simulink model "battery_pack"  (R2021a)
settings: Solver=VariableStepAuto  StartTime=0.0  StopTime=300  RelTol=1e-3
libraries: fl_lib x3, nesl_utility x3
settings Model: Creator=miche  LastModifiedBy=miche

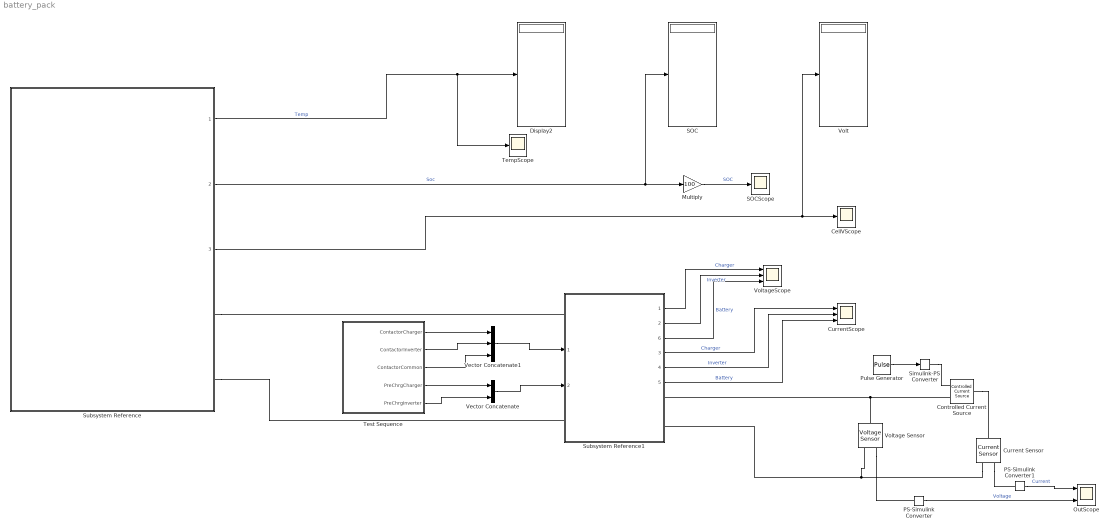
== system battery_pack ==
  CellVScope : Scope
  Controlled Current Source : fl_lib/Electrical/Electrical Sources/Controlled Current Source
  Current Sensor : fl_lib/Electrical/Electrical Sensors/Current Sensor
  CurrentScope : Scope  NumInputPorts=3
  Display2 : Display
  Multiply : Gain  Gain=100
  OutScope : Scope  NumInputPorts=2
  PS-Simulink Converter : nesl_utility/PS-Simulink Converter  PhysicalDomain=network_engine_domain  SubClassName=ps_output  LeftPortType=input  RightPortType=output  PseudoPeriodic=off  Frequencies=[]  Unit=inherit  AffineConversion=off
      settings: SourceProductBaseCode=PW,SS
  PS-Simulink Converter1 : nesl_utility/PS-Simulink Converter  PhysicalDomain=network_engine_domain  SubClassName=ps_output  LeftPortType=input  RightPortType=output  PseudoPeriodic=off  Frequencies=[]  Unit=inherit  AffineConversion=off
      settings: SourceProductBaseCode=PW,SS
  Pulse Generator : DiscretePulseGenerator  PulseType=Time based  Amplitude=22  Period=25  PulseWidth=30  PhaseDelay=100
  SOC : Display
  SOCScope : Scope
  Simulink-PS Converter : nesl_utility/Simulink-PS Converter  PhysicalDomain=network_engine_domain  SubClassName=ps_input  LeftPortType=input  RightPortType=output  PseudoPeriodic=off  Frequencies=[]  NoiseDistribution=none  NoiseParameters=[]  Unit=1  AffineConversion=off  FilteringAndDerivatives=provide  SimscapeFilterOrder=1  InputFilterTimeConstant=0.001  UdotUserProvided=0
      settings: SourceProductBaseCode=PW,SS
  Subsystem Reference : Subsystem  ReferencedSubsystem=battery_module
  Subsystem Reference1 : Subsystem  ReferencedSubsystem=contactor_module
      settings: PortSchema="{\"entries\":[{\"content\":{\"sides\":[{\"content\":{\"connectorIds\":[\"LConn1\",\"In1\",\"In2\",\"LConn2\"]},\"type\":\"ConnectorPlacement.EquallySpacedRectSide\",\"uuid\":\"2f432158-1751-4d2f-82af-aaaffea8bda9\"},{\"content\":{\"connectorIds\":[\"Out1\",\"Out2\",\"Out6\",\"Out3\",\"Out4\",\"Out5\",\"RConn2\",\"RConn1\",\"RConn3\"],\"side\":\"RIGHT\"},\"type\":\"ConnectorPlacement.EquallySpacedRectSide\",\"uuid\":\"cc9680cc-f41c-4952-901e-103b0367ee37\"},{\"content\":{\"connectorIds\":[],\"side\":\"TOP\"},\"type\":\"ConnectorPlacement.EquallySpacedRectSide\",\"uuid\":\"20ab27d2-aefa-496d-9589-3b1d932ebb8b\"}]},\"type\":\"ConnectorPlacement.EquallySpacedConnector\",\"uuid\":\"b0306086-ee48-4285-994d-c35b8b48ddfd\"}],\"packageUris\":[\"http://schema.mathworks.com/mf0/Connector/R2020b\"],\"version\":\"1.0\"}"
  TempScope : Scope
  Test Sequence : Test Sequence  TreatAsAtomicUnit=on
  Vector Concatenate : Concatenate
  Vector Concatenate1 : Concatenate  NumInputs=3
  Volt : Display
  Voltage Sensor : fl_lib/Electrical/Electrical Sensors/Voltage Sensor
  VoltageScope : Scope  NumInputPorts=3
  wires:
  Subsystem Reference1/2 -> VoltageScope/2  "Inverter"
  PS-Simulink Converter1/1 -> OutScope/1  "Current"
  Subsystem Reference1/1 -> VoltageScope/1  "Charger"
  PS-Simulink Converter/1 -> OutScope/2  "Voltage"
  Subsystem Reference/2 -> Multiply/1, SOC/1  "Soc"
  Multiply/1 -> SOCScope/1  "SOC"
  Subsystem Reference/1 -> TempScope/1, Display2/1  "Temp"
  Test Sequence/4(PreChrgCharger) -> Vector Concatenate/1
  Test Sequence/5(PreChrgInverter) -> Vector Concatenate/2
  Test Sequence/1(ContactorCharger) -> Vector Concatenate1/1
  Test Sequence/2(ContactorInverter) -> Vector Concatenate1/2
  Test Sequence/3(ContactorCommon) -> Vector Concatenate1/3
  Subsystem Reference1/6 -> VoltageScope/3  "Battery"
  Subsystem Reference1/3 -> CurrentScope/1  "Charger"
  Subsystem Reference1/4 -> CurrentScope/2  "Inverter"
  Subsystem Reference1/5 -> CurrentScope/3  "Battery"
  Subsystem Reference/3 -> CellVScope/1, Volt/1
  Vector Concatenate1/1 -> Subsystem Reference1/1
  Vector Concatenate/1 -> Subsystem Reference1/2
  Pulse Generator/1 -> Simulink-PS Converter/1
  connections:
  Voltage Sensor/RConn2 -- Current Sensor/RConn2 -- Subsystem Reference1/RConn3
  Voltage Sensor/RConn1 -- PS-Simulink Converter/LConn1
  Voltage Sensor/LConn1 -- Subsystem Reference1/RConn2 -- Controlled Current Source/RConn2
  Current Sensor/RConn1 -- PS-Simulink Converter1/LConn1
  Subsystem Reference/RConn2 -- Subsystem Reference1/LConn2
  Subsystem Reference/RConn1 -- Subsystem Reference1/LConn1
  Controlled Current Source/LConn1 -- Current Sensor/LConn1
  Simulink-PS Converter/RConn1 -- Controlled Current Source/RConn1

== stateflow chart battery_pack/Test Sequence ==
  state step_1
    ContactorCommon = 0;
    PreChrgCharger = 0;
    PreChrgInverter = 0;
    ContactorCharger = 0;
    ContactorInverter = 0;
  state step_2
    ContactorCommon = 1;
  state step_3
    PreChrgCharger = 1;
  state step_4
    PreChrgInverter = 1;
  state step_5
    ContactorCharger = 1;
  state step_6
    ContactorInverter = 1;
  state step_7
    PreChrgCharger = 0;
    ContactorCharger = 0;
    PreChrgInverter = 0;
  (default) -> step_1
  step_1 -> step_2 : [
      | true
      | ]
  step_2 -> step_3 : [
      | after(0.5, sec)
      | ]
  step_3 -> step_4 : [
      | after(10, sec)
      | ]
  step_4 -> step_5 : [
      | after(3, sec)
      | ]
  step_5 -> step_6 : [
      | after(5, sec)
      | ]
  step_6 -> step_7 : [
      | after(5, sec)
      | ]
  data: ContactorCharger output; ContactorInverter output; ContactorCommon output; PreChrgCharger output; PreChrgInverter output
